simulink model "UKF"  (Simulink 8.0)
settings: Solver=ode1  StartTime=0.0  StopTime=Inf  FixedStep=0.001  RelTol=1e-3
undefined symbols (not defined in the file or in its folder): alpha, beta, d_p1, d_p2, g, kappa, l_1, l_2, m_1, m_2, m_3, P, Q, R, T, x0
settings Model: Creator=Bosselmann  LastModifiedBy=Bosselmann  BufferReuse=off
settings OptimizationCC: BlockReduction=off  OptimizeBlockIOStorage=off  BufferReuse=off  ExpressionFolding=off  LocalBlockOutputs=off
settings HardwareCC: ProdIntDivRoundTo=Zero  ProdEndianess=BigEndian  ProdHWDeviceType=Generic->Custom  TargetIntDivRoundTo=Zero  TargetEndianess=BigEndian  TargetHWDeviceType=Generic->Custom
settings RTWCC: SystemTargetFile=rti1401.tlc  MakeCommand=make_rti  TemplateMakefile=rti1401.tmf  Description=dSPACE DS1401 Hardware Platform  ProcessScript=rti1401_make_rtw_hook
settings STFCustomTargetCC: CodeReplacementLibrary=ANSI_C  ParMdlRefBuildCompliant=on  GeneratePreprocessorConditionals=Disable all  MatFileLogging=on  SystemTargetFile=rti1401.tlc
settings GRTTargetCC: CompOptLevelCompliant=off  ConcurrentExecutionCompliant=off  CombineOutputUpdateFcns=off  GRTInterface=on
settings CustomProperty: DataType=RTWOptions_EnumType_C__Program Files (x86)_dSPACE RCPHIL 74_MATLAB_RTI_RTI1401_TLC_rti1401_1InitialSimState  Value=RUN
settings EnumStrPairs: String=RUN

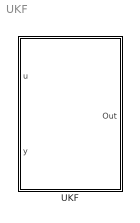
== system UKF ==
  UKF : Subsystem

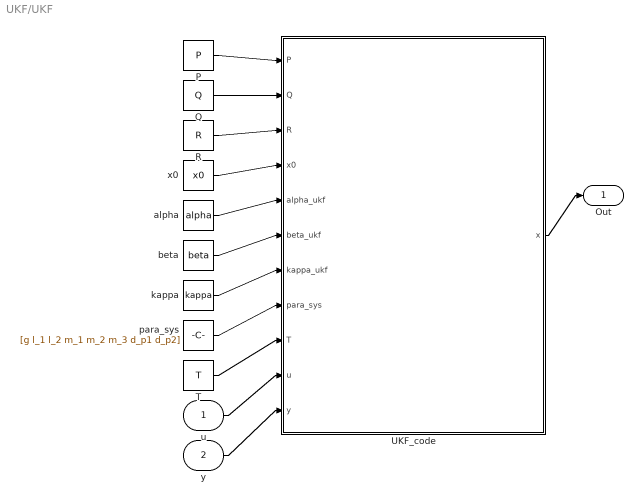
== system UKF/UKF ==
  u : Inport
  y : Inport  Port=2
  P : Constant  Value=P
  Q : Constant  Value=Q
  R : Constant  Value=R
  T : Constant  Value=T
  UKF_code : MATLAB Function  TreatAsAtomicUnit=on
  alpha : Constant  Value=alpha
  beta : Constant  Value=beta
  kappa : Constant  Value=kappa
  para_sys : Constant  Value=[g l_1 l_2 m_1 m_2 m_3 d_p1 d_p2]
  x0 : Constant  Value=x0
  Out : Outport
  wires:
  P/1 -> UKF_code/1(P)
  Q/1 -> UKF_code/2(Q)
  R/1 -> UKF_code/3(R)
  x0/1 -> UKF_code/4(x0)
  alpha/1 -> UKF_code/5(alpha_ukf)
  beta/1 -> UKF_code/6(beta_ukf)
  kappa/1 -> UKF_code/7(kappa_ukf)
  para_sys/1 -> UKF_code/8(para_sys)
  T/1 -> UKF_code/9(T)
  u/1 -> UKF_code/10(u)
  y/1 -> UKF_code/11(y)
  UKF_code/1(x) -> Out/1

== matlab function UKF/UKF_code ==
  data: P input double; Q input double; R input double; x0 input double; alpha_ukf input double; beta_ukf input double; kappa_ukf input double; para_sys input double; T input double; u input double; y input double; x output double
function x = unscented_kalman_filter(P, Q, R, x0, alpha_ukf, beta_ukf, kappa_ukf, para_sys, T, u, y)
% Unscented Kalman Filter (UKF) fuer nichtlineare Systeme
% Das UKF praediziert den Zustand eines nichtliniearen Systems durch
% Mittelung sog. Sigma Punkte. Dazu werden 2n+1 Sigmapunkte (moegliche
% Zustaende des Systems) mittels Kovarianzmatrix P berechnet und fuer jeden
% Sigmapunkt mithilfe der Zustandsgleichung ein neuer Zustand praediziert.
% Diese werden gewichtet gemittelt und mit deren Hilfe die neuen
% Kovarianzmatrizen, die Rueckfuehrmatrix K und die Zustaende ermittelt.
% Weitere Infos unter
% http://www.agnld.uni-potsdam.de/~shw/TSA/Tools/UKF/node4.html
% http://cslu.cse.ogi.edu/nsel/ukf/node6.html
%
% Tipp: kappa meist zu 0 waehlen, alpha sehr klein bspw. 0.001, beta bei
% Gaussverteilung = 2
% -alpha bestimmt die Streuung der Sigma-Punkte um den Mittelwert
% -beta wird benutzt, um Wissen ueber die Verteilung aufzunehmen
% -kappa ist ein sekundaerer skalierender Parameter, der gewoehnlich 
% gleich 0 oder 3-n gesetzt wird
%
% Vorlage von Matthias Dagen, September 2009, veraendert durch David
% Klinkenbuss

persistent x_p P_p x0_sig x_sig W_m W_c

% Parameter

g = para_sys(1);
l_1 = para_sys(2);
l_2 = para_sys(3);
m_1 = para_sys(4);
m_2 = para_sys(5);
m_3 = para_sys(6);
d_p1 = para_sys(7);
d_p2 = para_sys(8);

n_ukf  = 4;     % Laenge von f(x)
o_ukf = 1;      % Anzahl der zurueckgefuehrten Variablen

if isempty(x_p) || isempty(P_p) || isempty(x0_sig) || isempty(x_sig) || isempty(W_m) || isempty(W_c)
    x_p = x0;
    P_p = P;
    x0_sig = zeros(n_ukf,2*n_ukf+1);
    x_sig  = zeros(n_ukf,2*n_ukf+1);
    W_m = zeros(1,2*n_ukf+1);
    W_c = zeros(1,2*n_ukf+1);
    x = x_p;
else

%% Parameter-Initialization
lambda_ukf = (alpha_ukf^2)*(n_ukf+kappa_ukf)-n_ukf;

%% Weight calculation
W_m(1,1) = lambda_ukf/(n_ukf+lambda_ukf);
W_c(1,1) = lambda_ukf/(n_ukf+lambda_ukf)+1-alpha_ukf^2+beta_ukf;
for i=2:2*n_ukf+1
    W_m(1,i) = 1/(2*(n_ukf+lambda_ukf));
    W_c(1,i) = 1/(2*(n_ukf+lambda_ukf));
end

%% 2n+1 Sigma Points calculation

P_an = (sqrt(n_ukf+lambda_ukf).*chol(P_p))'; % Wurzelmatrix mittels Cholesky-Zerlegung
x0_sig(:,1) = x_p;
for i=2:n_ukf+1
    x0_sig(:,i)     = x_p + P_an(:,i-1);
    x0_sig(:,n_ukf+i)   = x_p - P_an(:,i-1);
end

%% Unscented Kalman filter time update equations
for i = 1:(2*n_ukf+1)


 x_1 = x0_sig(1,i);
 x_2 = x0_sig(2,i);
 x_3 = x0_sig(3,i);
 x_4 = x0_sig(4,i);

x_sig(:,i) = [x_1 + T*x_2;x_2 + (T*(12*d_p2*l_2*x_4 - 12*d_p1*l_2*x_2 - 12*d_p2*l_2*x_2 - cos(x_1 - x_3)*(18*d_p2*l_1*x_2 - 18*d_p2*l_1*x_4 + 9*l_1*l_2*m_2*u*cos(x_3) + 9*g*l_1*l_2*m_2*sin(x_3) + 9*l_1^2*l_2*m_2*x_2^2*sin(x_1 - x_3)) + 6*l_1*l_2*m_1*u*cos(x_1) + 12*l_1*l_2*m_2*u*cos(x_1) + 12*l_1*l_2*m_3*u*cos(x_1) + 6*g*l_1*l_2*m_1*sin(x_1) + 12*g*l_1*l_2*m_2*sin(x_1) + 12*g*l_1*l_2*m_3*sin(x_1) - 6*l_1*l_2^2*m_2*x_4^2*sin(x_1 - x_3)))/(l_1^2*l_2*(4*m_1 + 12*m_2 + 12*m_3 - 9*m_2*cos(x_1 - x_3)^2));x_3 + T*x_4;x_4 + (T*(sin(x_1 - x_3)*(36*l_1^2*l_2*m_2^2*x_2^2 + 12*l_1^2*l_2*m_1*m_2*x_2^2 + 36*l_1^2*l_2*m_2*m_3*x_2^2) + 24*d_p2*l_1*m_1*x_2 + 72*d_p2*l_1*m_2*x_2 - 24*d_p2*l_1*m_1*x_4 + 72*d_p2*l_1*m_3*x_2 - 72*d_p2*l_1*m_2*x_4 - 72*d_p2*l_1*m_3*x_4 + 36*d_p1*l_2*m_2*x_2*cos(x_1 - x_3) + 36*d_p2*l_2*m_2*x_2*cos(x_1 - x_3) - 36*d_p2*l_2*m_2*x_4*cos(x_1 - x_3) + 18*l_1*l_2*m_2^2*u*cos(x_3) + 18*g*l_1*l_2*m_2^2*sin(x_3) + 9*l_1*l_2^2*m_2^2*x_4^2*sin(2*x_1 - 2*x_3) - 18*l_1*l_2*m_2^2*u*cos(2*x_1 - x_3) - 18*g*l_1*l_2*m_2^2*sin(2*x_1 - x_3) + 3*l_1*l_2*m_1*m_2*u*cos(x_3) + 18*l_1*l_2*m_2*m_3*u*cos(x_3) + 3*g*l_1*l_2*m_1*m_2*sin(x_3) + 18*g*l_1*l_2*m_2*m_3*sin(x_3) - 9*l_1*l_2*m_1*m_2*u*cos(2*x_1 - x_3) - 18*l_1*l_2*m_2*m_3*u*cos(2*x_1 - x_3) - 9*g*l_1*l_2*m_1*m_2*sin(2*x_1 - x_3) - 18*g*l_1*l_2*m_2*m_3*sin(2*x_1 - x_3)))/(l_1*l_2^2*m_2*(8*m_1 + 15*m_2 + 24*m_3 - 9*m_2*cos(2*x_1 - 2*x_3)))];

end
y_sig= [1 0 0 0] * x_sig;
% Prediction, weighted sum
x_p  = x_sig * W_m';
y_  = y_sig * W_m';
%P_p calculation
P_p = P_p .* 0;
for i=1:(2*n_ukf+1)
    P_p = P_p + ((x_sig(:,i) - x_p) * (x_sig(:,i) - x_p)' .* W_c(1,i));
end
P_p  = P_p + Q;

%% Unscented Kalman filter measurement update equations
% Pyy calculation
P_yy = zeros(o_ukf,o_ukf);
for i=1:(2*n_ukf+1)
    P_yy = P_yy + ((y_sig(:,i) - y_) * (y_sig(:,i) - y_)' .* W_c(1,i));
end
P_yy = P_yy + R;
% Pxy calculation
P_xy = zeros(n_ukf,o_ukf);
for i=1:(2*n_ukf+1)
    P_xy = P_xy+((x_sig(:,i)-x_p)*(y_sig(:,i)-y_)'.*W_c(1,i));
end
% Kalman Gain
K  = P_xy/(P_yy);
P_p = P_p - (K * P_yy * K');
x  = x_p +  K * ( y - y_);
x_p = x;
end
